simulink model "Part_2"  (R2021b)
settings: Solver=VariableStepAuto  StartTime=0.0  StopTime=10.0  RelTol=1e-3
settings Model: Creator=Bader Gamal  LastModifiedBy=Bader Gamal

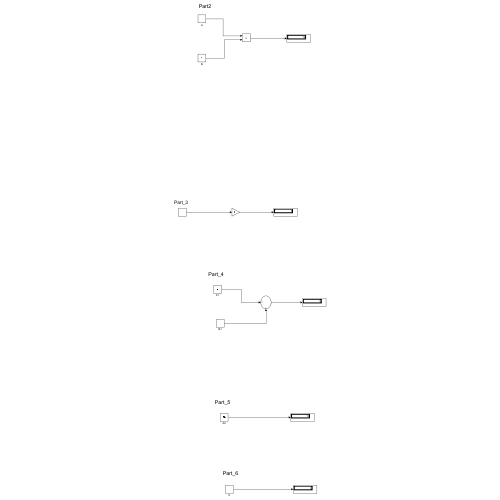
[thumbnail: Simulink's stored preview of the top-level diagram]
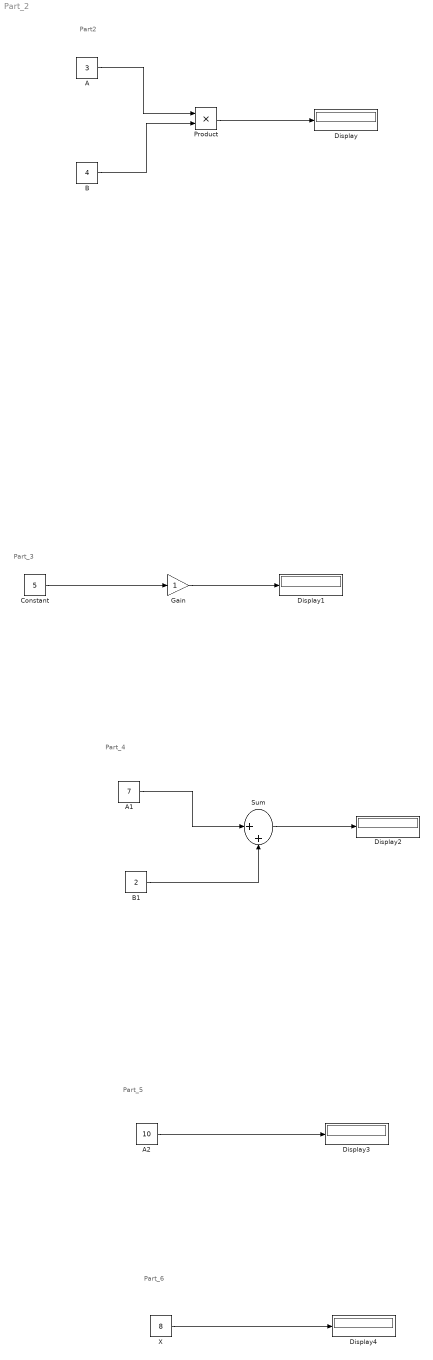
== system Part_2 ==
  note: Part_4
  note: Part_3
  note: Part2
  note: Part_5
  note: Part_6
  A : Constant  Value=3
  A1 : Constant  Value=7
  A2 : Constant  Value=10
  B : Constant  Value=4
  B1 : Constant  Value=2
  Constant : Constant  Value=5
  Display{,1..4} (5 alike) : Display
  Gain : Gain
  Product : Product
  Sum : Sum  Inputs=|++
  X : Constant  Value=8
  wires:
  Constant/1 -> Gain/1
  Gain/1 -> Display1/1
  B/1 -> Product/2
  A/1 -> Product/1
  Product/1 -> Display/1
  A1/1 -> Sum/1
  B1/1 -> Sum/2
  Sum/1 -> Display2/1
  A2/1 -> Display3/1
  X/1 -> Display4/1
